simulink model "control_system"  (R2020b)
settings: Solver=FixedStepAuto  StartTime=0.0  StopTime=t_sim  FixedStep=Ts  RelTol=1e-2
values from neighbouring files (symbols this model uses):
  Hp = 10    [main_script.m]
  InitPosX = -2.4980e+03    (= -2498)    [main_script.m]
  InitPosY = -650.5503    [main_script.m]
  InitVelX = V0*cosd(InitYaw)    [main_script.m]
  InitVelY = V0*sind(InitYaw)    [main_script.m]
  InitYaw = 21    [main_script.m]
  lr = 1.592    [main_script.m]
  m = 1625    [main_script.m]
  Ts = 0.1    [main_script.m]
  V0 = 25    [main_script.m]
libraries: neural x856, simulink x1, autolibshared x1, drivingscenarioandsensors x1
(part 24 of 40)

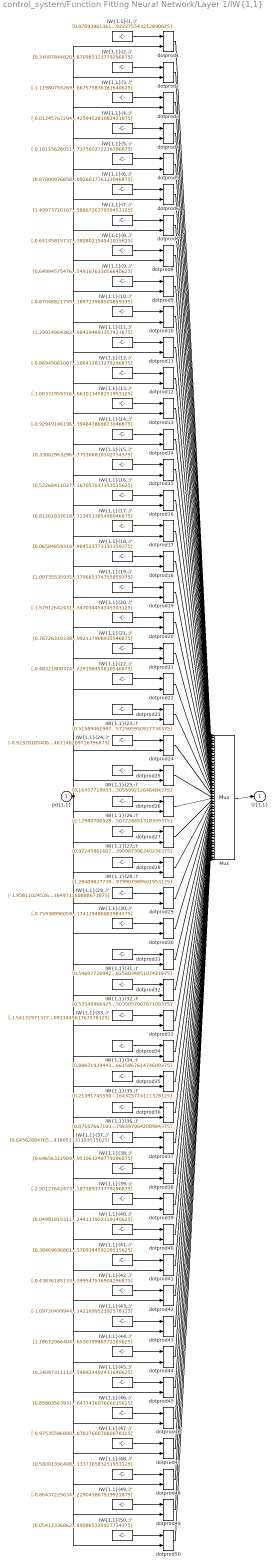
== system control_system/Function Fitting Neural Network/Layer 1/IW{1,1} ==
  "pd{1,1}" : Inport  PortDimensions=9  SampleTime=0.1
      mask Display: e = 0.06;c1 = [120 230 180]/255;c2 = ([120 230 180]+0)/(256+128);c3 = ([120 230 180]+128)/(256+128);patch([0 1 1 0],[0 0 1 1],c1);patch([0 1 1 1-e 1-e 0+e],[0 0 1 1-e 0+e 0+e],c2);patch([0 0 1 1-e 0+e 0+e],[0 1 1 1-e 1-e 0+e],c3);plot([0 1 1 0 0],[0 0 1 1 0]);
  "IW{1,1}(1,:)'" : Constant  Value=[0.97093961361378278152045595561503432691097259521484375;-0.28039871116987102883655325058498419821262359619140625;0.3851709807844587718506090823211707174777984619140625;-0.5135982842823201277582256807363592088222503662109375;1.1922160293525363439215425387374125421047210693359375;-2.639146237323939825358820598921738564968109130859375;-0.2450864019114529501752741680320468731224536895751953125;1.7910155270211147726655553924501873552799224853515625;-0.3880197795036404162516419091843999922275543212890625]
      mask Display: e = 0.06;c1 = [120 150 230]/255;c2 = ([120 150 230]+0)/383;c3 = ([120 150 230]+128)/383;patch([0 1 1 0],[0 0 1 1],c1);patch([0 1 1 1-e 1-e 0+e],[0 0 1 1-e 0+e 0+e],c2);patch([0 0 1 1-e 0+e 0+e],[0 1 1 1-e 1-e 0+e],c3);plot([0 1 1 0 0],[0 0 1 1 0]);disp('Weights');
  "IW{1,1}(10,:)'" : Constant  Value=[-0.87046821799074114434091598013765178620815277099609375;-0.270184812964925857858844437942025251686573028564453125;-0.43314155483321326034484854972106404602527618408203125;-1.590306799106527169129776666522957384586334228515625;-1.1862880482407736071337467365083284676074981689453125;-0.9888726559320486497739466358325444161891937255859375;-0.96914646726430786483064139247289858758449554443359375;-1.04056527906724483045763918198645114898681640625;-0.1494792541584611667015991542939445935189723968505859375]
      mask Display: e = 0.06;c1 = [120 150 230]/255;c2 = ([120 150 230]+0)/383;c3 = ([120 150 230]+128)/383;patch([0 1 1 0],[0 0 1 1],c1);patch([0 1 1 1-e 1-e 0+e],[0 0 1 1-e 0+e 0+e],c2);patch([0 0 1 1-e 0+e 0+e],[0 1 1 1-e 1-e 0+e],c3);plot([0 1 1 0 0],[0 0 1 1 0]);disp('Weights');
  "IW{1,1}(11,:)'" : Constant  Value=[1.2991496438276917135823396165505982935428619384765625;-0.25365900898659543560853535382193513214588165283203125;0.4141726146470963154655464677489362657070159912109375;1.210520214599590804738227234338410198688507080078125;-1.190198107523747328428953551338054239749908447265625;-1.869803133332969213853402834502048790454864501953125;-0.07196017006668704862892838036714238114655017852783203125;2.999680955949197258547656019800342619419097900390625;-0.059496514302423912645689796363512868992984294891357421875]
      mask Display: e = 0.06;c1 = [120 150 230]/255;c2 = ([120 150 230]+0)/383;c3 = ([120 150 230]+128)/383;patch([0 1 1 0],[0 0 1 1],c1);patch([0 1 1 1-e 1-e 0+e],[0 0 1 1-e 0+e 0+e],c2);patch([0 0 1 1-e 0+e 0+e],[0 1 1 1-e 1-e 0+e],c3);plot([0 1 1 0 0],[0 0 1 1 0]);disp('Weights');
  "IW{1,1}(12,:)'" : Constant  Value=[-0.86945061007791668572508569923229515552520751953125;0.290923752853725459122102847686619497835636138916015625;0.95093882023071019116144952931790612637996673583984375;-1.9489697439161499659121545846574008464813232421875;-1.519461066101597257471667035133577883243560791015625;1.2565348140057448489415037329308688640594482421875;0.933333136450000377948299501440487802028656005859375;1.0652420654480423412024947538156993687152862548828125;0.049200942200943502402576967824643361382186412811279296875]
      mask Display: e = 0.06;c1 = [120 150 230]/255;c2 = ([120 150 230]+0)/383;c3 = ([120 150 230]+128)/383;patch([0 1 1 0],[0 0 1 1],c1);patch([0 1 1 1-e 1-e 0+e],[0 0 1 1-e 0+e 0+e],c2);patch([0 0 1 1-e 0+e 0+e],[0 1 1 1-e 1-e 0+e],c3);plot([0 1 1 0 0],[0 0 1 1 0]);disp('Weights');
  "IW{1,1}(13,:)'" : Constant  Value=[-1.003319593162952827469780459068715572357177734375;0.67810826771338283958101555981556884944438934326171875;-0.61043188678200721586364352333475835621356964111328125;0.70916334762463384411290689968154765665531158447265625;-0.5759983806607589240655897810938768088817596435546875;2.2490521260628018040961251244880259037017822265625;0.72014281285539805121942436016979627311229705810546875;0.63362322182121577629487774174776859581470489501953125;-1.126765513624864656350155200925655663013458251953125]
      mask Display: e = 0.06;c1 = [120 150 230]/255;c2 = ([120 150 230]+0)/383;c3 = ([120 150 230]+128)/383;patch([0 1 1 0],[0 0 1 1],c1);patch([0 1 1 1-e 1-e 0+e],[0 0 1 1-e 0+e 0+e],c2);patch([0 0 1 1-e 0+e 0+e],[0 1 1 1-e 1-e 0+e],c3);plot([0 1 1 0 0],[0 0 1 1 0]);disp('Weights');
  "IW{1,1}(14,:)'" : Constant  Value=[-0.92949146196026521948851950583048164844512939453125;-1.1429665455757758163457538103102706372737884521484375;1.0519091572919772037408847609185613691806793212890625;-1.14525233529797532128213788382709026336669921875;-0.981528358989009586110796590219251811504364013671875;0.9179910649476141770719550549983978271484375;-1.318360733295090625460943556390702724456787109375;1.1479820287018203117668235790915787220001220703125;-0.44393580226848594616484433572622947394847869873046875]
      mask Display: e = 0.06;c1 = [120 150 230]/255;c2 = ([120 150 230]+0)/383;c3 = ([120 150 230]+128)/383;patch([0 1 1 0],[0 0 1 1],c1);patch([0 1 1 1-e 1-e 0+e],[0 0 1 1-e 0+e 0+e],c2);patch([0 0 1 1-e 0+e 0+e],[0 1 1 1-e 1-e 0+e],c3);plot([0 1 1 0 0],[0 0 1 1 0]);disp('Weights');
  "IW{1,1}(15,:)'" : Constant  Value=[0.338029632961837911420133195861126296222209930419921875;0.64599406331379516377211302824434824287891387939453125;0.83768969923422087475728403660468757152557373046875;0.1967697974008914829635585874711978249251842498779296875;1.222289857737168805584815345355309545993804931640625;0.408573274266887775940659821571898646652698516845703125;-1.3644966924852666156908753691823221743106842041015625;-0.63673533425992301371110215768567286431789398193359375;-0.438606434078379459062801970503642223775386810302734375]
      mask Display: e = 0.06;c1 = [120 150 230]/255;c2 = ([120 150 230]+0)/383;c3 = ([120 150 230]+128)/383;patch([0 1 1 0],[0 0 1 1],c1);patch([0 1 1 1-e 1-e 0+e],[0 0 1 1-e 0+e 0+e],c2);patch([0 0 1 1-e 0+e 0+e],[0 1 1 1-e 1-e 0+e],c3);plot([0 1 1 0 0],[0 0 1 1 0]);disp('Weights');
  "IW{1,1}(16,:)'" : Constant  Value=[0.52268411027939698509925392500008456408977508544921875;0.56795133558729860023817082037567161023616790771484375;-0.82591672355761158730302895492059178650379180908203125;-0.370849859231966172412597870788886211812496185302734375;-0.85030315566211955857767179622896946966648101806640625;-2.594022559460632759709142192150466144084930419921875;-1.1273055818606410038995591094135306775569915771484375;1.727361799815982923433921314426697790622711181640625;0.29135109056686714357198297875584103167057037353515625]
      mask Display: e = 0.06;c1 = [120 150 230]/255;c2 = ([120 150 230]+0)/383;c3 = ([120 150 230]+128)/383;patch([0 1 1 0],[0 0 1 1],c1);patch([0 1 1 1-e 1-e 0+e],[0 0 1 1-e 0+e 0+e],c2);patch([0 0 1 1-e 0+e 0+e],[0 1 1 1-e 1-e 0+e],c3);plot([0 1 1 0 0],[0 0 1 1 0]);disp('Weights');
  "IW{1,1}(17,:)'" : Constant  Value=[0.81261837618960386375732696251361630856990814208984375;0.11240683240479144855417104054140509106218814849853515625;-0.5429613049158803494975700232316739857196807861328125;-0.06735020182903361796178387521649710834026336669921875;0.39746836699794185765455267755896784365177154541015625;-2.289745303179948177074720661039464175701141357421875;-2.36823235121522213120215383241884410381317138671875;-0.01920417466123570948699494920219876803457736968994140625;-0.78248758849519528535410017866524867713451385498046875]
      mask Display: e = 0.06;c1 = [120 150 230]/255;c2 = ([120 150 230]+0)/383;c3 = ([120 150 230]+128)/383;patch([0 1 1 0],[0 0 1 1],c1);patch([0 1 1 1-e 1-e 0+e],[0 0 1 1-e 0+e 0+e],c2);patch([0 0 1 1-e 0+e 0+e],[0 1 1 1-e 1-e 0+e],c3);plot([0 1 1 0 0],[0 0 1 1 0]);disp('Weights');
  "IW{1,1}(18,:)'" : Constant  Value=[0.06584859319073210759398762093042023479938507080078125;0.62491571055994155070578699451289139688014984130859375;0.7990170181207203459194943206966854631900787353515625;-0.75432588489251550800673840058152563869953155517578125;0.13406440645860673299694099114276468753814697265625;-1.33187501082899029114514632965438067913055419921875;-0.1785974939056451937791081263640080578625202178955078125;1.7897623143730687633734532937523908913135528564453125;-1.1695125433076183352198995635262690484523773193359375]
      mask Display: e = 0.06;c1 = [120 150 230]/255;c2 = ([120 150 230]+0)/383;c3 = ([120 150 230]+128)/383;patch([0 1 1 0],[0 0 1 1],c1);patch([0 1 1 1-e 1-e 0+e],[0 0 1 1-e 0+e 0+e],c2);patch([0 0 1 1-e 0+e 0+e],[0 1 1 1-e 1-e 0+e],c3);plot([0 1 1 0 0],[0 0 1 1 0]);disp('Weights');
  "IW{1,1}(19,:)'" : Constant  Value=[1.0973553593516409687680379647645168006420135498046875;-0.57538307796085741419034320642822422087192535400390625;-0.6837986697134279534537881772848777472972869873046875;-0.94680710579524696157704966026358306407928466796875;0.88746712770898217303994215399143286049365997314453125;-1.381451882267370923074167876620776951313018798828125;1.0848135377034520132610850851051509380340576171875;0.261632884446667990374635337502695620059967041015625;-0.414726180288912116278510211486718617379665374755859375]
      mask Display: e = 0.06;c1 = [120 150 230]/255;c2 = ([120 150 230]+0)/383;c3 = ([120 150 230]+128)/383;patch([0 1 1 0],[0 0 1 1],c1);patch([0 1 1 1-e 1-e 0+e],[0 0 1 1-e 0+e 0+e],c2);patch([0 0 1 1-e 0+e 0+e],[0 1 1 1-e 1-e 0+e],c3);plot([0 1 1 0 0],[0 0 1 1 0]);disp('Weights');
  "IW{1,1}(2,:)'" : Constant  Value=[0.340078448202071947914504335130914114415645599365234375;0.61152168668360207259837579840677790343761444091796875;1.1084410511733011617252486757934093475341796875;-0.62989834861553595235506008975789882242679595947265625;-0.58042049387658967152248123966273851692676544189453125;-2.466934744743214391604624324827454984188079833984375;-1.2023642587252083568927218948374502360820770263671875;1.0666891089756165289514910909929312765598297119140625;-0.5594774025453748134140141701209358870983123779296875]
      mask Display: e = 0.06;c1 = [120 150 230]/255;c2 = ([120 150 230]+0)/383;c3 = ([120 150 230]+128)/383;patch([0 1 1 0],[0 0 1 1],c1);patch([0 1 1 1-e 1-e 0+e],[0 0 1 1-e 0+e 0+e],c2);patch([0 0 1 1-e 0+e 0+e],[0 1 1 1-e 1-e 0+e],c3);plot([0 1 1 0 0],[0 0 1 1 0]);disp('Weights');
  "IW{1,1}(20,:)'" : Constant  Value=[-1.57912642431413541288520718808285892009735107421875;0.61409549742207769629231961516779847443103790283203125;1.1686478953490155863192967444774694740772247314453125;-1.1848793747106174389926991352695040404796600341796875;-1.239529920774651738923921584500931203365325927734375;1.809648206205790810230382703593932092189788818359375;-0.20529698998786205521582814981229603290557861328125;3.47991716679978413395701863919384777545928955078125;-0.1594062963675073885116972860487294383347034454345703125]
      mask Display: e = 0.06;c1 = [120 150 230]/255;c2 = ([120 150 230]+0)/383;c3 = ([120 150 230]+128)/383;patch([0 1 1 0],[0 0 1 1],c1);patch([0 1 1 1-e 1-e 0+e],[0 0 1 1-e 0+e 0+e],c2);patch([0 0 1 1-e 0+e 0+e],[0 1 1 1-e 1-e 0+e],c3);plot([0 1 1 0 0],[0 0 1 1 0]);disp('Weights');
  "IW{1,1}(21,:)'" : Constant  Value=[0.7672631033851498028042215082678012549877166748046875;-0.458108958975613156372475032185320742428302764892578125;-0.59701861006420475774802980595268309116363525390625;-0.519756145505974931353421197854913771152496337890625;0.54766554871049688557604895322583615779876708984375;2.312553685817124726753490904229693114757537841796875;0.11270256966186241454064287381697795353829860687255859375;-1.7338209275897338290661764403921552002429962158203125;-0.26046106414641723159064667925122193992137908935546875]
      mask Display: e = 0.06;c1 = [120 150 230]/255;c2 = ([120 150 230]+0)/383;c3 = ([120 150 230]+128)/383;patch([0 1 1 0],[0 0 1 1],c1);patch([0 1 1 1-e 1-e 0+e],[0 0 1 1-e 0+e 0+e],c2);patch([0 0 1 1-e 0+e 0+e],[0 1 1 1-e 1-e 0+e],c3);plot([0 1 1 0 0],[0 0 1 1 0]);disp('Weights');
  "IW{1,1}(22,:)'" : Constant  Value=[-0.48321808374106300920658441100385971367359161376953125;-0.65067428012154138183831264541368000209331512451171875;0.403709011817810381472781955380924046039581298828125;-0.97435270094193315859598669703700579702854156494140625;0.94881194703902094200742567409179173409938812255859375;-0.3906213358896533094366532168351113796234130859375;-0.477089342851166831049880556747666560113430023193359375;1.0488331207768648578593229103717021644115447998046875;1.275361389429331193667849220219068229198455810546875]
      mask Display: e = 0.06;c1 = [120 150 230]/255;c2 = ([120 150 230]+0)/383;c3 = ([120 150 230]+128)/383;patch([0 1 1 0],[0 0 1 1],c1);patch([0 1 1 1-e 1-e 0+e],[0 0 1 1-e 0+e 0+e],c2);patch([0 0 1 1-e 0+e 0+e],[0 1 1 1-e 1-e 0+e],c3);plot([0 1 1 0 0],[0 0 1 1 0]);disp('Weights');
  "IW{1,1}(23,:)'" : Constant  Value=[0.51589461997649888047590138739906251430511474609375;0.87745139464428933973039193006115965545177459716796875;-0.032613147418183031922556125437040464021265506744384765625;-0.03530138783985899142425779473342117853462696075439453125;1.190955473178289647506744586280547082424163818359375;2.559180139348819604805385097279213368892669677734375;0.1537049497733080360983848322575795464217662811279296875;1.8488371095364704022045998499379493296146392822265625;0.82838062523518285473755895509384572505950927734375]
      mask Display: e = 0.06;c1 = [120 150 230]/255;c2 = ([120 150 230]+0)/383;c3 = ([120 150 230]+128)/383;patch([0 1 1 0],[0 0 1 1],c1);patch([0 1 1 1-e 1-e 0+e],[0 0 1 1-e 0+e 0+e],c2);patch([0 0 1 1-e 0+e 0+e],[0 1 1 1-e 1-e 0+e],c3);plot([0 1 1 0 0],[0 0 1 1 0]);disp('Weights');
  "IW{1,1}(24,:)'" : Constant  Value=[-0.92320185406252708304464249522425234317779541015625;0.1589026907972997670892567612099810503423213958740234375;1.336759816706434289557137162773869931697845458984375;-0.5072895852030858687697900677449069917201995849609375;-0.83277156532756346773993527676793746650218963623046875;-0.58680259947876234338792755806935019791126251220703125;0.98203138856916927235118919270462356507778167724609375;0.1387309905135986343172049828353920020163059234619140625;-1.498732567071687338255969734746031463146209716796875]
      mask Display: e = 0.06;c1 = [120 150 230]/255;c2 = ([120 150 230]+0)/383;c3 = ([120 150 230]+128)/383;patch([0 1 1 0],[0 0 1 1],c1);patch([0 1 1 1-e 1-e 0+e],[0 0 1 1-e 0+e 0+e],c2);patch([0 0 1 1-e 0+e 0+e],[0 1 1 1-e 1-e 0+e],c3);plot([0 1 1 0 0],[0 0 1 1 0]);disp('Weights');
  "IW{1,1}(25,:)'" : Constant  Value=[0.164577189330164352920604642349644564092159271240234375;0.84274510322094287051442051961203105747699737548828125;1.0828171979316782991276113534695468842983245849609375;-0.95362354157796136444602552728611044585704803466796875;-0.65823826889210146351416597099159844219684600830078125;-0.342232460185585007916841959740850143134593963623046875;-1.31956634967429931037941059912554919719696044921875;-1.3632672320762908579894201466231606900691986083984375;-0.58440502948554795548119500381289981305599212646484375]
      mask Display: e = 0.06;c1 = [120 150 230]/255;c2 = ([120 150 230]+0)/383;c3 = ([120 150 230]+128)/383;patch([0 1 1 0],[0 0 1 1],c1);patch([0 1 1 1-e 1-e 0+e],[0 0 1 1-e 0+e 0+e],c2);patch([0 0 1 1-e 0+e 0+e],[0 1 1 1-e 1-e 0+e],c3);plot([0 1 1 0 0],[0 0 1 1 0]);disp('Weights');
  "IW{1,1}(26,:)'" : Constant  Value=[2.129807065288331191510451390058733522891998291015625;-0.107603565378774523875193835920072160661220550537109375;0.3974472819784342636495466649648733437061309814453125;0.2283305403113514431279185146195231936872005462646484375;-1.17135151038194607053810614161193370819091796875;-0.09955161999984911413985599892839672975242137908935546875;-0.69388861218623343329880981400492601096630096435546875;1.5917799632123525999105595474247820675373077392578125;0.07577917958936251918711235475711873732507228851318359375]
      mask Display: e = 0.06;c1 = [120 150 230]/255;c2 = ([120 150 230]+0)/383;c3 = ([120 150 230]+128)/383;patch([0 1 1 0],[0 0 1 1],c1);patch([0 1 1 1-e 1-e 0+e],[0 0 1 1-e 0+e 0+e],c2);patch([0 0 1 1-e 0+e 0+e],[0 1 1 1-e 1-e 0+e],c3);plot([0 1 1 0 0],[0 0 1 1 0]);disp('Weights');
  "IW{1,1}(27,:)'" : Constant  Value=[0.972458616076971704700326881720684468746185302734375;0.80071168334724396320467576515511609613895416259765625;-0.69820535755774570940701551080564968287944793701171875;-0.5759124849266401557912331554689444601535797119140625;-0.128118934045561239098987016404862515628337860107421875;-1.478205651886735250144511155667714774608612060546875;0.0077068368952901457336057688962682732380926609039306640625;-0.998042389125082696210711219464428722858428955078125;-0.714100168764340903493348378106020390987396240234375]
      mask Display: e = 0.06;c1 = [120 150 230]/255;c2 = ([120 150 230]+0)/383;c3 = ([120 150 230]+128)/383;patch([0 1 1 0],[0 0 1 1],c1);patch([0 1 1 1-e 1-e 0+e],[0 0 1 1-e 0+e 0+e],c2);patch([0 0 1 1-e 0+e 0+e],[0 1 1 1-e 1-e 0+e],c3);plot([0 1 1 0 0],[0 0 1 1 0]);disp('Weights');
  "IW{1,1}(28,:)'" : Constant  Value=[1.2940982773928013660480473845382221043109893798828125;-0.375899268560394850258177257273928262293338775634765625;0.52795145605138327216110383233171887695789337158203125;0.8920181642611628713979143867618404328823089599609375;-0.7564801989411666927054511688766069710254669189453125;-0.93565270712781833939430953250848688185214996337890625;1.2753434908208323150802243617363274097442626953125;-2.1016583865335274339258830877952277660369873046875;-0.96344937374039407718129268687334842979907989501953125]
      mask Display: e = 0.06;c1 = [120 150 230]/255;c2 = ([120 150 230]+0)/383;c3 = ([120 150 230]+128)/383;patch([0 1 1 0],[0 0 1 1],c1);patch([0 1 1 1-e 1-e 0+e],[0 0 1 1-e 0+e 0+e],c2);patch([0 0 1 1-e 0+e 0+e],[0 1 1 1-e 1-e 0+e],c3);plot([0 1 1 0 0],[0 0 1 1 0]);disp('Weights');
  "IW{1,1}(29,:)'" : Constant  Value=[-1.9581102452695378079994270592578686773777008056640625;-0.51412525497394268025885821771225892007350921630859375;0.20836627953751907238455487458850257098674774169921875;-0.67867145203121570506965554159251041710376739501953125;-0.73024135157208525104266527705476619303226470947265625;-1.352942975596346020239479912561364471912384033203125;0.396568187054604115449052414987818337976932525634765625;1.317863646844906089228288692538626492023468017578125;-1.97243397611674264879866314004175364971160888671875]
      mask Display: e = 0.06;c1 = [120 150 230]/255;c2 = ([120 150 230]+0)/383;c3 = ([120 150 230]+128)/383;patch([0 1 1 0],[0 0 1 1],c1);patch([0 1 1 1-e 1-e 0+e],[0 0 1 1-e 0+e 0+e],c2);patch([0 0 1 1-e 0+e 0+e],[0 1 1 1-e 1-e 0+e],c3);plot([0 1 1 0 0],[0 0 1 1 0]);disp('Weights');
  "IW{1,1}(3,:)'" : Constant  Value=[-1.1198075526975130866702556886593811213970184326171875;-0.20507969346321497372542808079742826521396636962890625;-0.289346350572056376648788500460796058177947998046875;0.720249732554860688793496592552401125431060791015625;-0.331892783688242765105513853995944373309612274169921875;-1.233167629340175874830265456694178283214569091796875;0.6903163444130335779647111849044449627399444580078125;-0.347081239760978821351500300806947052478790283203125;0.90246068479395946670962302960106171667575836181640625]
      mask Display: e = 0.06;c1 = [120 150 230]/255;c2 = ([120 150 230]+0)/383;c3 = ([120 150 230]+128)/383;patch([0 1 1 0],[0 0 1 1],c1);patch([0 1 1 1-e 1-e 0+e],[0 0 1 1-e 0+e 0+e],c2);patch([0 0 1 1-e 0+e 0+e],[0 1 1 1-e 1-e 0+e],c3);plot([0 1 1 0 0],[0 0 1 1 0]);disp('Weights');
  "IW{1,1}(30,:)'" : Constant  Value=[-0.759389960599416991016141764703206717967987060546875;0.2840216328908475862391469490830786526203155517578125;0.94276840524974547808056968278833664953708648681640625;0.97160631832165711418980436064884997904300689697265625;-0.58575567778431592014243278754292987287044525146484375;0.8372478811272221488337663686252199113368988037109375;-0.71782872175648304580164449362200684845447540283203125;-0.436041221124511102491538849790231324732303619384765625;1.1028566606177123698984132715850137174129486083984375]
      mask Display: e = 0.06;c1 = [120 150 230]/255;c2 = ([120 150 230]+0)/383;c3 = ([120 150 230]+128)/383;patch([0 1 1 0],[0 0 1 1],c1);patch([0 1 1 1-e 1-e 0+e],[0 0 1 1-e 0+e 0+e],c2);patch([0 0 1 1-e 0+e 0+e],[0 1 1 1-e 1-e 0+e],c3);plot([0 1 1 0 0],[0 0 1 1 0]);disp('Weights');
  "IW{1,1}(31,:)'" : Constant  Value=[0.5460772094207744231653123279102146625518798828125;0.460953363760126411108331012655980885028839111328125;-0.2115703979530784983875690841159666888415813446044921875;0.69504683404170808369570977447438053786754608154296875;0.8940914594258568826035116217099130153656005859375;-1.1341484239892289931361801791354082524776458740234375;-0.78412324798395693914443427274818532168865203857421875;0.458013400742934617682067255373112857341766357421875;-0.87559191277812054021723042751546017825603485107421875]
      mask Display: e = 0.06;c1 = [120 150 230]/255;c2 = ([120 150 230]+0)/383;c3 = ([120 150 230]+128)/383;patch([0 1 1 0],[0 0 1 1],c1);patch([0 1 1 1-e 1-e 0+e],[0 0 1 1-e 0+e 0+e],c2);patch([0 0 1 1-e 0+e 0+e],[0 1 1 1-e 1-e 0+e],c3);plot([0 1 1 0 0],[0 0 1 1 0]);disp('Weights');
  "IW{1,1}(32,:)'" : Constant  Value=[0.5354996642529721295744593589915893971920013427734375;1.2428883524386815651041615637950599193572998046875;0.228676873276494274644932147566578350961208343505859375;-0.74924171147733920061995149808353744447231292724609375;-0.16774896417198348341770497427205555140972137451171875;-0.196043865385012450186508203842095099389553070068359375;0.91169744811784669824561433415510691702365875244140625;2.152452022970312128791192662902176380157470703125;-0.6080750191048698294338237246847711503505706787109375]
      mask Display: e = 0.06;c1 = [120 150 230]/255;c2 = ([120 150 230]+0)/383;c3 = ([120 150 230]+128)/383;patch([0 1 1 0],[0 0 1 1],c1);patch([0 1 1 1-e 1-e 0+e],[0 0 1 1-e 0+e 0+e],c2);patch([0 0 1 1-e 0+e 0+e],[0 1 1 1-e 1-e 0+e],c3);plot([0 1 1 0 0],[0 0 1 1 0]);disp('Weights');
  "IW{1,1}(33,:)'" : Constant  Value=[-1.54132971377970395820966587052680552005767822265625;-0.25072633293704693624448509581270627677440643310546875;0.159123795845034277096630148662370629608631134033203125;0.842653609044052398502344658481888473033905029296875;-0.10573959777820692018668324863028828985989093780517578125;-0.032706632404859485585557621334373834542930126190185546875;1.010366189247158263952997003798373043537139892578125;0.59077516492751780408099193664384074509143829345703125;-1.4585530146121705730166695502703078091144561767578125]
      mask Display: e = 0.06;c1 = [120 150 230]/255;c2 = ([120 150 230]+0)/383;c3 = ([120 150 230]+128)/383;patch([0 1 1 0],[0 0 1 1],c1);patch([0 1 1 1-e 1-e 0+e],[0 0 1 1-e 0+e 0+e],c2);patch([0 0 1 1-e 0+e 0+e],[0 1 1 1-e 1-e 0+e],c3);plot([0 1 1 0 0],[0 0 1 1 0]);disp('Weights');
  "IW{1,1}(34,:)'" : Constant  Value=[0.88671928443622871629514747837674804031848907470703125;-0.120878905322355512108600805731839500367641448974609375;-0.4035700109378390632031141649349592626094818115234375;-0.92663839697876160261813538454589433968067169189453125;-1.0135453088708319402400093167671002447605133056640625;-1.173695312179412919562082606717012822628021240234375;-0.5347377780826312321238447111682035028934478759765625;0.127868778308200814475270590264699421823024749755859375;0.91237645222570085135060935499495826661586761474609375]
      mask Display: e = 0.06;c1 = [120 150 230]/255;c2 = ([120 150 230]+0)/383;c3 = ([120 150 230]+128)/383;patch([0 1 1 0],[0 0 1 1],c1);patch([0 1 1 1-e 1-e 0+e],[0 0 1 1-e 0+e 0+e],c2);patch([0 0 1 1-e 0+e 0+e],[0 1 1 1-e 1-e 0+e],c3);plot([0 1 1 0 0],[0 0 1 1 0]);disp('Weights');
  "IW{1,1}(35,:)'" : Constant  Value=[0.2139174555065020688626731271142489276826381683349609375;-0.94378848270968995759488961994065903127193450927734375;-0.77573954351650609151391790874185971915721893310546875;0.832673531343797179715693346224725246429443359375;0.5534326111105565271230943835689686238765716552734375;0.483365499823072308771543248440138995647430419921875;-1.0535779933159463706004999039578251540660858154296875;0.1461396229710316685412863080273382365703582763671875;-1.2308373766330504839316972720553167164325714111328125]
      mask Display: e = 0.06;c1 = [120 150 230]/255;c2 = ([120 150 230]+0)/383;c3 = ([120 150 230]+128)/383;patch([0 1 1 0],[0 0 1 1],c1);patch([0 1 1 1-e 1-e 0+e],[0 0 1 1-e 0+e 0+e],c2);patch([0 0 1 1-e 0+e 0+e],[0 1 1 1-e 1-e 0+e],c3);plot([0 1 1 0 0],[0 0 1 1 0]);disp('Weights');
  "IW{1,1}(36,:)'" : Constant  Value=[0.071076671037090921601020454545505344867706298828125;0.664168033627640763683075419976375997066497802734375;1.8291748250620083471318366719060577452182769775390625;0.3820678757705116002085787840769626200199127197265625;0.59425875284591211933360455077490769326686859130859375;-0.76784223084368019573986430259537883102893829345703125;-0.655048484051070634137658998952247202396392822265625;-2.145149871234647509510296004009433090686798095703125;-1.4557464670865216671558073358028195798397064208984375]
      mask Display: e = 0.06;c1 = [120 150 230]/255;c2 = ([120 150 230]+0)/383;c3 = ([120 150 230]+128)/383;patch([0 1 1 0],[0 0 1 1],c1);patch([0 1 1 1-e 1-e 0+e],[0 0 1 1-e 0+e 0+e],c2);patch([0 0 1 1-e 0+e 0+e],[0 1 1 1-e 1-e 0+e],c3);plot([0 1 1 0 0],[0 0 1 1 0]);disp('Weights');
  "IW{1,1}(37,:)'" : Constant  Value=[0.6456288476568701195645871848682872951030731201171875;-0.65799923001170046443775163425016216933727264404296875;0.311582392682186404275768154548131860792636871337890625;-0.89148107540302323759107139267143793404102325439453125;-0.50996951927726552611375154810957610607147216796875;-0.51393130227626360184700615718611516058444976806640625;1.078650466544016861547561347833834588527679443359375;-0.73422117746091630774429859229712747037410736083984375;-0.95155828196638891913750057938159443438053131103515625]
      mask Display: e = 0.06;c1 = [120 150 230]/255;c2 = ([120 150 230]+0)/383;c3 = ([120 150 230]+128)/383;patch([0 1 1 0],[0 0 1 1],c1);patch([0 1 1 1-e 1-e 0+e],[0 0 1 1-e 0+e 0+e],c2);patch([0 0 1 1-e 0+e 0+e],[0 1 1 1-e 1-e 0+e],c3);plot([0 1 1 0 0],[0 0 1 1 0]);disp('Weights');
  "IW{1,1}(38,:)'" : Constant  Value=[0.6965632290952339378264923652750439941883087158203125;-1.047869280408078029864782365621067583560943603515625;0.10172333557136960247024859427256160415709018707275390625;-0.65579721068447904830378547558211721479892730712890625;0.476182384031906769106257115709013305604457855224609375;-0.454386696705189108147493470823974348604679107666015625;-0.67927572398451141477693226988776586949825286865234375;-0.9500830060727418757693385487073101103305816650390625;1.5277450016389397813298955952632240951061248779296875]
      mask Display: e = 0.06;c1 = [120 150 230]/255;c2 = ([120 150 230]+0)/383;c3 = ([120 150 230]+128)/383;patch([0 1 1 0],[0 0 1 1],c1);patch([0 1 1 1-e 1-e 0+e],[0 0 1 1-e 0+e 0+e],c2);patch([0 0 1 1-e 0+e 0+e],[0 1 1 1-e 1-e 0+e],c3);plot([0 1 1 0 0],[0 0 1 1 0]);disp('Weights');
  "IW{1,1}(39,:)'" : Constant  Value=[-2.501276424736501358125906335772015154361724853515625;-1.54408584292858819253524416126310825347900390625;0.53902133932544804562070339670754037797451019287109375;-2.47586042911307036007428905577398836612701416015625;-1.58608884985863429761820952990092337131500244140625;-1.8602628445853326422110285420785658061504364013671875;-0.79149527778107697795206831870018504559993743896484375;0.52007634687461756772819398975116200745105743408203125;0.65448293706638682731835388040053658187389373779296875]
      mask Display: e = 0.06;c1 = [120 150 230]/255;c2 = ([120 150 230]+0)/383;c3 = ([120 150 230]+128)/383;patch([0 1 1 0],[0 0 1 1],c1);patch([0 1 1 1-e 1-e 0+e],[0 0 1 1-e 0+e 0+e],c2);patch([0 0 1 1-e 0+e 0+e],[0 1 1 1-e 1-e 0+e],c3);plot([0 1 1 0 0],[0 0 1 1 0]);disp('Weights');
  "IW{1,1}(4,:)'" : Constant  Value=[-0.01245767294369288895328207189550084876827895641326904296875;-0.411636498589336874420752110381727106869220733642578125;0.2343696751666357325216694107439252547919750213623046875;0.151189163508950119574336667938041500747203826904296875;-0.55434305624034874160344088522833772003650665283203125;-1.8245528196456344272036176334950141608715057373046875;-0.463261564773732870126110583441914059221744537353515625;1.46145194046994930658911471255123615264892578125;2.084219744558360343233971434528939425945281982421875]
      mask Display: e = 0.06;c1 = [120 150 230]/255;c2 = ([120 150 230]+0)/383;c3 = ([120 150 230]+128)/383;patch([0 1 1 0],[0 0 1 1],c1);patch([0 1 1 1-e 1-e 0+e],[0 0 1 1-e 0+e 0+e],c2);patch([0 0 1 1-e 0+e 0+e],[0 1 1 1-e 1-e 0+e],c3);plot([0 1 1 0 0],[0 0 1 1 0]);disp('Weights');
  "IW{1,1}(40,:)'" : Constant  Value=[0.0499181531106483167281595569875207729637622833251953125;1.0051321772202594928558028186671435832977294921875;-0.270173244365803422173399894745671190321445465087890625;-1.3445729513710948932470046202070079743862152099609375;-0.2261562490857440266278644003250519745051860809326171875;1.9768896600832850385387473579612560570240020751953125;-0.96232631804396728814054995382321067154407501220703125;0.251580362866357931661553948288201354444026947021484375;1.15310724398443031901706490316428244113922119140625]
      mask Display: e = 0.06;c1 = [120 150 230]/255;c2 = ([120 150 230]+0)/383;c3 = ([120 150 230]+128)/383;patch([0 1 1 0],[0 0 1 1],c1);patch([0 1 1 1-e 1-e 0+e],[0 0 1 1-e 0+e 0+e],c2);patch([0 0 1 1-e 0+e 0+e],[0 1 1 1-e 1-e 0+e],c3);plot([0 1 1 0 0],[0 0 1 1 0]);disp('Weights');
  "IW{1,1}(41,:)'" : Constant  Value=[0.38469696861631141882043039004202000796794891357421875;-0.2480663135903987959185457157218479551374912261962890625;-1.1349625028722438724315679792198352515697479248046875;-0.7068117105996154503344541808473877608776092529296875;1.0943346055495497548548655686317943036556243896484375;0.217780452520371980984492665811558254063129425048828125;-0.8727094143813707294299319983110763132572174072265625;0.63296503258427627702786821828340180218219757080078125;0.30266956728881366789352114210487343370914459228515625]
      mask Display: e = 0.06;c1 = [120 150 230]/255;c2 = ([120 150 230]+0)/383;c3 = ([120 150 230]+128)/383;patch([0 1 1 0],[0 0 1 1],c1);patch([0 1 1 1-e 1-e 0+e],[0 0 1 1-e 0+e 0+e],c2);patch([0 0 1 1-e 0+e 0+e],[0 1 1 1-e 1-e 0+e],c3);plot([0 1 1 0 0],[0 0 1 1 0]);disp('Weights');
  "IW{1,1}(42,:)'" : Constant  Value=[-0.4383618513340941102995884648407809436321258544921875;-0.57418463271939013115030547851347364485263824462890625;-0.66654353817884282040751031672698445618152618408203125;-0.28523372835698623806166551730711944401264190673828125;0.97122275204309260754342858490417711436748504638671875;0.53016822367742044708194271152024157345294952392578125;-0.5308267262522157192705662964726798236370086669921875;-1.204748771676599883306835181429050862789154052734375;0.52152863773203594899285917563247494399547576904296875]
      mask Display: e = 0.06;c1 = [120 150 230]/255;c2 = ([120 150 230]+0)/383;c3 = ([120 150 230]+128)/383;patch([0 1 1 0],[0 0 1 1],c1);patch([0 1 1 1-e 1-e 0+e],[0 0 1 1-e 0+e 0+e],c2);patch([0 0 1 1-e 0+e 0+e],[0 1 1 1-e 1-e 0+e],c3);plot([0 1 1 0 0],[0 0 1 1 0]);disp('Weights');
  "IW{1,1}(43,:)'" : Constant  Value=[-1.097204999444521877904890061472542583942413330078125;-0.06095196396622311330038002097353455610573291778564453125;-1.2088855521526815639532514978782273828983306884765625;-0.5664032353071044578740611541434191167354583740234375;1.039673180341422753514279975206591188907623291015625;-1.90933576109207781001941839349456131458282470703125;0.55569237221125933334775481853284873068332672119140625;-0.425995643434998016996217984342365525662899017333984375;-0.032752510386764743799403731827624142169952392578125]
      mask Display: e = 0.06;c1 = [120 150 230]/255;c2 = ([120 150 230]+0)/383;c3 = ([120 150 230]+128)/383;patch([0 1 1 0],[0 0 1 1],c1);patch([0 1 1 1-e 1-e 0+e],[0 0 1 1-e 0+e 0+e],c2);patch([0 0 1 1-e 0+e 0+e],[0 1 1 1-e 1-e 0+e],c3);plot([0 1 1 0 0],[0 0 1 1 0]);disp('Weights');
  "IW{1,1}(44,:)'" : Constant  Value=[1.1867206640414227347690712122130207717418670654296875;-0.51641328540057163110077453893609344959259033203125;-1.029288781821291909324145308346487581729888916015625;0.1761470882763403189574802354400162585079669952392578125;-0.817240127933413607053125815582461655139923095703125;-0.29719985756557354417140004443353973329067230224609375;-0.376403083287819573143906382028944790363311767578125;0.7379027639523181303360388483270071446895599365234375;0.522499458097746671825234443531371653079986572265625]
      mask Display: e = 0.06;c1 = [120 150 230]/255;c2 = ([120 150 230]+0)/383;c3 = ([120 150 230]+128)/383;patch([0 1 1 0],[0 0 1 1],c1);patch([0 1 1 1-e 1-e 0+e],[0 0 1 1-e 0+e 0+e],c2);patch([0 0 1 1-e 0+e 0+e],[0 1 1 1-e 1-e 0+e],c3);plot([0 1 1 0 0],[0 0 1 1 0]);disp('Weights');
  "IW{1,1}(45,:)'" : Constant  Value=[0.240973111125132255505576495124842040240764617919921875;0.377473013572193483167183103432762436568737030029296875;0.416452240351548874652820586561574600636959075927734375;-0.166501497516372831686481958968215622007846832275390625;-1.834082844585235960721547598950564861297607421875;3.3892664252582758166454368620179593563079833984375;-0.0748724992258840982284340270780376158654689788818359375;-0.444894164332242880721679512134869582951068878173828125;-0.14343269040447526041504033855744637548923492431640625]
      mask Display: e = 0.06;c1 = [120 150 230]/255;c2 = ([120 150 230]+0)/383;c3 = ([120 150 230]+128)/383;patch([0 1 1 0],[0 0 1 1],c1);patch([0 1 1 1-e 1-e 0+e],[0 0 1 1-e 0+e 0+e],c2);patch([0 0 1 1-e 0+e 0+e],[0 1 1 1-e 1-e 0+e],c3);plot([0 1 1 0 0],[0 0 1 1 0]);disp('Weights');
  "IW{1,1}(46,:)'" : Constant  Value=[0.85803563931209880788486543679027818143367767333984375;-0.63961669920042718562314121300005353987216949462890625;-1.8790915052350367631106564658693969249725341796875;-0.124242937280011067624485576743609271943569183349609375;0.434112243372880957092974085753667168319225311279296875;-0.07580442069907462887545790408694301731884479522705078125;-0.20038215540647164036869298797682859003543853759765625;-0.4380871196766673580924589259666390717029571533203125;0.404227687614099606694395561135024763643741607666015625]
      mask Display: e = 0.06;c1 = [120 150 230]/255;c2 = ([120 150 230]+0)/383;c3 = ([120 150 230]+128)/383;patch([0 1 1 0],[0 0 1 1],c1);patch([0 1 1 1-e 1-e 0+e],[0 0 1 1-e 0+e 0+e],c2);patch([0 0 1 1-e 0+e 0+e],[0 1 1 1-e 1-e 0+e],c3);plot([0 1 1 0 0],[0 0 1 1 0]);disp('Weights');
  "IW{1,1}(47,:)'" : Constant  Value=[-0.97535586890674874638307301211170852184295654296875;-0.299335465871109318580778335672221146523952484130859375;-0.28790071651083148918104370750370435416698455810546875;-1.707306349052662763909893328673206269741058349609375;-0.424632458065148321590953628401621244847774505615234375;-1.7167520343473963162495010692509822547435760498046875;-1.3155488353961513059431354122352786362171173095703125;-0.73148446576655212769679792472743429243564605712890625;-0.90745028209644396088862094984506256878376007080078125]
      mask Display: e = 0.06;c1 = [120 150 230]/255;c2 = ([120 150 230]+0)/383;c3 = ([120 150 230]+128)/383;patch([0 1 1 0],[0 0 1 1],c1);patch([0 1 1 1-e 1-e 0+e],[0 0 1 1-e 0+e 0+e],c2);patch([0 0 1 1-e 0+e 0+e],[0 1 1 1-e 1-e 0+e],c3);plot([0 1 1 0 0],[0 0 1 1 0]);disp('Weights');
  "IW{1,1}(48,:)'" : Constant  Value=[0.58001396408077654509582998798578046262264251708984375;-1.519046330984501924632468217168934643268585205078125;-0.56950056035899765394248106531449593603610992431640625;0.324523052716408189066754630403011105954647064208984375;-1.27647180417102301674958653165958821773529052734375;0.77654160714141429178170028535532765090465545654296875;0.65278250713822616457804315359680913388729095458984375;0.71456416558735924571266195926000364124774932861328125;0.96951647422195297298941341068712063133716583251953125]
      mask Display: e = 0.06;c1 = [120 150 230]/255;c2 = ([120 150 230]+0)/383;c3 = ([120 150 230]+128)/383;patch([0 1 1 0],[0 0 1 1],c1);patch([0 1 1 1-e 1-e 0+e],[0 0 1 1-e 0+e 0+e],c2);patch([0 0 1 1-e 0+e 0+e],[0 1 1 1-e 1-e 0+e],c3);plot([0 1 1 0 0],[0 0 1 1 0]);disp('Weights');
  "IW{1,1}(49,:)'" : Constant  Value=[-0.86437225634516712258204051977372728288173675537109375;0.98171685428277866147794838980189524590969085693359375;0.019456189134307556865000066181892179884016513824462890625;0.93457076825025009458869362788391299545764923095703125;-0.716132009219719645187751666526310145854949951171875;0.1391102844191524356975975251771160401403903961181640625;0.6054396940132116267108131069107912480831146240234375;0.97250202007511610258205791978980414569377899169921875;0.479736723293402611556501824452425353229045867919921875]
      mask Display: e = 0.06;c1 = [120 150 230]/255;c2 = ([120 150 230]+0)/383;c3 = ([120 150 230]+128)/383;patch([0 1 1 0],[0 0 1 1],c1);patch([0 1 1 1-e 1-e 0+e],[0 0 1 1-e 0+e 0+e],c2);patch([0 0 1 1-e 0+e 0+e],[0 1 1 1-e 1-e 0+e],c3);plot([0 1 1 0 0],[0 0 1 1 0]);disp('Weights');
  "IW{1,1}(5,:)'" : Constant  Value=[-0.181156260513459788086265689344145357608795166015625;0.6201558592768481315005146825569681823253631591796875;-0.92873871939931651464661399586475454270839691162109375;-0.14649962329492416390763764866278506815433502197265625;-0.723763893029772287235346084344200789928436279296875;-0.175056695761272529399121822279994376003742218017578125;-1.1039947092468300748890897011733613908290863037109375;0.84960381390248074229276653568376787006855010986328125;-0.72889227291211244885715814234572462737560272216796875]
      mask Display: e = 0.06;c1 = [120 150 230]/255;c2 = ([120 150 230]+0)/383;c3 = ([120 150 230]+128)/383;patch([0 1 1 0],[0 0 1 1],c1);patch([0 1 1 1-e 1-e 0+e],[0 0 1 1-e 0+e 0+e],c2);patch([0 0 1 1-e 0+e 0+e],[0 1 1 1-e 1-e 0+e],c3);plot([0 1 1 0 0],[0 0 1 1 0]);disp('Weights');
  "IW{1,1}(50,:)'" : Constant  Value=[0.054123368625048372260177842463235720060765743255615234375;0.74976423299714334280707817015354521572589874267578125;-1.1783432860728193514177064571413211524486541748046875;-0.69060360291757250106314813820063136518001556396484375;0.86871111050459293156933426871546544134616851806640625;-0.406972539882097306129793423679075203835964202880859375;0.031903777161261158423766204350613406859338283538818359375;0.56555808722542566524538187877624295651912689208984375;-1.14937646256341707839965238235890865325927734375]
      mask Display: e = 0.06;c1 = [120 150 230]/255;c2 = ([120 150 230]+0)/383;c3 = ([120 150 230]+128)/383;patch([0 1 1 0],[0 0 1 1],c1);patch([0 1 1 1-e 1-e 0+e],[0 0 1 1-e 0+e 0+e],c2);patch([0 0 1 1-e 0+e 0+e],[0 1 1 1-e 1-e 0+e],c3);plot([0 1 1 0 0],[0 0 1 1 0]);disp('Weights');
  "IW{1,1}(6,:)'" : Constant  Value=[0.87000976858961343030074431226239539682865142822265625;0.7110350945318122395377713473862968385219573974609375;-1.2759595695332432985225068478030152618885040283203125;1.2054218240237222214972234723973087966442108154296875;0.83833544909682855550414615208865143358707427978515625;1.5559780003582430740749487085849978029727935791015625;0.698202525683534691580689468537457287311553955078125;-0.17286948979518290681056669200188480317592620849609375;-0.373453768756931647754271352823707275092601776123046875]
      mask Display: e = 0.06;c1 = [120 150 230]/255;c2 = ([120 150 230]+0)/383;c3 = ([120 150 230]+128)/383;patch([0 1 1 0],[0 0 1 1],c1);patch([0 1 1 1-e 1-e 0+e],[0 0 1 1-e 0+e 0+e],c2);patch([0 0 1 1-e 0+e 0+e],[0 1 1 1-e 1-e 0+e],c3);plot([0 1 1 0 0],[0 0 1 1 0]);disp('Weights');
  "IW{1,1}(7,:)'" : Constant  Value=[1.4997372016747945178138934352318756282329559326171875;-0.418144995355191839703223877222626470029354095458984375;-0.223661784933861351731820832355879247188568115234375;0.9646418008850810021925781256868503987789154052734375;0.58275331566434107610774617569404654204845428466796875;1.4086511278745266206868791414308361709117889404296875;0.66061304729803682622701899163075722754001617431640625;-0.85347821356929298719506959969294257462024688720703125;0.564640016963342095124289699015207588672637939453125]
      mask Display: e = 0.06;c1 = [120 150 230]/255;c2 = ([120 150 230]+0)/383;c3 = ([120 150 230]+128)/383;patch([0 1 1 0],[0 0 1 1],c1);patch([0 1 1 1-e 1-e 0+e],[0 0 1 1-e 0+e 0+e],c2);patch([0 0 1 1-e 0+e 0+e],[0 1 1 1-e 1-e 0+e],c3);plot([0 1 1 0 0],[0 0 1 1 0]);disp('Weights');
  "IW{1,1}(8,:)'" : Constant  Value=[-0.64145815737887346141832267676363699138164520263671875;-1.1466409303196909430511141181341372430324554443359375;-0.376513844193542668303820164510398171842098236083984375;-0.354876733680442424390122369004529900848865509033203125;0.39032632476723494452386375996866263449192047119140625;1.1144230146539382264592177307349629700183868408203125;-0.99474015016140437950298291980288922786712646484375;1.34246851661036092906442718231119215488433837890625;-0.53861982069599945166515908567816950380802154541015625]
      mask Display: e = 0.06;c1 = [120 150 230]/255;c2 = ([120 150 230]+0)/383;c3 = ([120 150 230]+128)/383;patch([0 1 1 0],[0 0 1 1],c1);patch([0 1 1 1-e 1-e 0+e],[0 0 1 1-e 0+e 0+e],c2);patch([0 0 1 1-e 0+e 0+e],[0 1 1 1-e 1-e 0+e],c3);plot([0 1 1 0 0],[0 0 1 1 0]);disp('Weights');
  "IW{1,1}(9,:)'" : Constant  Value=[0.6499457547620723918413432329543866217136383056640625;0.87866119494201611050954170423210598528385162353515625;-1.01929567913466723183546491782180964946746826171875;-1.0428089589739835130188794209971092641353607177734375;0.68443113420214041209277411326183937489986419677734375;0.3412573356422889947481280614738352596759796142578125;0.59969312005255159814254284356138668954372406005859375;-1.1777031620542992573774654374574311077594757080078125;-0.96768538118119951096929298728355206549167633056640625]
      mask Display: e = 0.06;c1 = [120 150 230]/255;c2 = ([120 150 230]+0)/383;c3 = ([120 150 230]+128)/383;patch([0 1 1 0],[0 0 1 1],c1);patch([0 1 1 1-e 1-e 0+e],[0 0 1 1-e 0+e 0+e],c2);patch([0 0 1 1-e 0+e 0+e],[0 1 1 1-e 1-e 0+e],c3);plot([0 1 1 0 0],[0 0 1 1 0]);disp('Weights');
  Mux : Mux  Inputs=50
      mask Display: e = 0.06;c1 = [120 150 230]/255;c2 = ([120 150 230]+0)/383;c3 = ([120 150 230]+128)/383;patch([0 1 1 0],[0 0 1 1],c1);patch([0 1 1 1-e 1-e 0+e],[0 0 1 1-e 0+e 0+e],c2);patch([0 0 1 1-e 0+e 0+e],[0 1 1 1-e 1-e 0+e],c3);plot([0 1 1 0 0],[0 0 1 1 0]);disp('Mux');
  dotprod{1..50} (50 alike) : neural/Weight Functions/dotprod
  "iz{1,1}" : Outport
      mask Display: e = 0.06;c1 = [120 230 180]/255;c2 = ([120 230 180]+0)/(256+128);c3 = ([120 230 180]+128)/(256+128);patch([0 1 1 0],[0 0 1 1],c1);patch([0 1 1 1-e 1-e 0+e],[0 0 1 1-e 0+e 0+e],c2);patch([0 0 1 1-e 0+e 0+e],[0 1 1 1-e 1-e 0+e],c3);plot([0 1 1 0 0],[0 0 1 1 0]);
  wires:
  "IW{1,1}(1,:)'"/1 -> dotprod1/1
  "pd{1,1}"/1 -> dotprod1/2, dotprod2/2, dotprod3/2, dotprod4/2, dotprod5/2, dotprod6/2, dotprod7/2, dotprod8/2, dotprod9/2, dotprod10/2, dotprod11/2, dotprod12/2, dotprod13/2, dotprod14/2, dotprod15/2, dotprod16/2, dotprod17/2, dotprod18/2, dotprod19/2, dotprod20/2, dotprod21/2, dotprod22/2, dotprod23/2, dotprod24/2, dotprod25/2, dotprod26/2, dotprod27/2, dotprod28/2, dotprod29/2, dotprod30/2, dotprod31/2, dotprod32/2, dotprod33/2, dotprod34/2, dotprod35/2, dotprod36/2, dotprod37/2, dotprod38/2, dotprod39/2, dotprod40/2, dotprod41/2, dotprod42/2, dotprod43/2, dotprod44/2, dotprod45/2, dotprod46/2, dotprod47/2, dotprod48/2, dotprod49/2, dotprod50/2
  dotprod1/1 -> Mux/1
  "IW{1,1}(2,:)'"/1 -> dotprod2/1
  dotprod2/1 -> Mux/2
  "IW{1,1}(3,:)'"/1 -> dotprod3/1
  dotprod3/1 -> Mux/3
  "IW{1,1}(4,:)'"/1 -> dotprod4/1
  dotprod4/1 -> Mux/4
  "IW{1,1}(5,:)'"/1 -> dotprod5/1
  dotprod5/1 -> Mux/5
  "IW{1,1}(6,:)'"/1 -> dotprod6/1
  dotprod6/1 -> Mux/6
  "IW{1,1}(7,:)'"/1 -> dotprod7/1
  dotprod7/1 -> Mux/7
  "IW{1,1}(8,:)'"/1 -> dotprod8/1
  dotprod8/1 -> Mux/8
  "IW{1,1}(9,:)'"/1 -> dotprod9/1
  dotprod9/1 -> Mux/9
  "IW{1,1}(10,:)'"/1 -> dotprod10/1
  dotprod10/1 -> Mux/10
  "IW{1,1}(11,:)'"/1 -> dotprod11/1
  dotprod11/1 -> Mux/11
  "IW{1,1}(12,:)'"/1 -> dotprod12/1
  dotprod12/1 -> Mux/12
  "IW{1,1}(13,:)'"/1 -> dotprod13/1
  dotprod13/1 -> Mux/13
  "IW{1,1}(14,:)'"/1 -> dotprod14/1
  dotprod14/1 -> Mux/14
  "IW{1,1}(15,:)'"/1 -> dotprod15/1
  dotprod15/1 -> Mux/15
  "IW{1,1}(16,:)'"/1 -> dotprod16/1
  dotprod16/1 -> Mux/16
  "IW{1,1}(17,:)'"/1 -> dotprod17/1
  dotprod17/1 -> Mux/17
  "IW{1,1}(18,:)'"/1 -> dotprod18/1
  dotprod18/1 -> Mux/18
  "IW{1,1}(19,:)'"/1 -> dotprod19/1
  dotprod19/1 -> Mux/19
  "IW{1,1}(20,:)'"/1 -> dotprod20/1
  dotprod20/1 -> Mux/20
  "IW{1,1}(21,:)'"/1 -> dotprod21/1
  dotprod21/1 -> Mux/21
  "IW{1,1}(22,:)'"/1 -> dotprod22/1
  dotprod22/1 -> Mux/22
  "IW{1,1}(23,:)'"/1 -> dotprod23/1
  dotprod23/1 -> Mux/23
  "IW{1,1}(24,:)'"/1 -> dotprod24/1
  dotprod24/1 -> Mux/24
  "IW{1,1}(25,:)'"/1 -> dotprod25/1
  dotprod25/1 -> Mux/25
  "IW{1,1}(26,:)'"/1 -> dotprod26/1
  dotprod26/1 -> Mux/26
  "IW{1,1}(27,:)'"/1 -> dotprod27/1
  dotprod27/1 -> Mux/27
  "IW{1,1}(28,:)'"/1 -> dotprod28/1
  dotprod28/1 -> Mux/28
  "IW{1,1}(29,:)'"/1 -> dotprod29/1
  dotprod29/1 -> Mux/29
  "IW{1,1}(30,:)'"/1 -> dotprod30/1
  dotprod30/1 -> Mux/30
  "IW{1,1}(31,:)'"/1 -> dotprod31/1
  dotprod31/1 -> Mux/31
  "IW{1,1}(32,:)'"/1 -> dotprod32/1
  dotprod32/1 -> Mux/32
  "IW{1,1}(33,:)'"/1 -> dotprod33/1
  dotprod33/1 -> Mux/33
  "IW{1,1}(34,:)'"/1 -> dotprod34/1
  dotprod34/1 -> Mux/34
  "IW{1,1}(35,:)'"/1 -> dotprod35/1
  dotprod35/1 -> Mux/35
  "IW{1,1}(36,:)'"/1 -> dotprod36/1
  dotprod36/1 -> Mux/36
  "IW{1,1}(37,:)'"/1 -> dotprod37/1
  dotprod37/1 -> Mux/37
  "IW{1,1}(38,:)'"/1 -> dotprod38/1
  dotprod38/1 -> Mux/38
  "IW{1,1}(39,:)'"/1 -> dotprod39/1
  dotprod39/1 -> Mux/39
  "IW{1,1}(40,:)'"/1 -> dotprod40/1
  dotprod40/1 -> Mux/40
  "IW{1,1}(41,:)'"/1 -> dotprod41/1
  dotprod41/1 -> Mux/41
  "IW{1,1}(42,:)'"/1 -> dotprod42/1
  dotprod42/1 -> Mux/42
  "IW{1,1}(43,:)'"/1 -> dotprod43/1
  dotprod43/1 -> Mux/43
  "IW{1,1}(44,:)'"/1 -> dotprod44/1
  dotprod44/1 -> Mux/44
  "IW{1,1}(45,:)'"/1 -> dotprod45/1
  dotprod45/1 -> Mux/45
  "IW{1,1}(46,:)'"/1 -> dotprod46/1
  dotprod46/1 -> Mux/46
  "IW{1,1}(47,:)'"/1 -> dotprod47/1
  dotprod47/1 -> Mux/47
  "IW{1,1}(48,:)'"/1 -> dotprod48/1
  dotprod48/1 -> Mux/48
  "IW{1,1}(49,:)'"/1 -> dotprod49/1
  dotprod49/1 -> Mux/49
  "IW{1,1}(50,:)'"/1 -> dotprod50/1
  dotprod50/1 -> Mux/50
  Mux/1 -> "iz{1,1}"/1

== system control_system/Function Fitting Neural Network/Layer 2/Delays 1 ==
  "p{2}" : Inport  PortDimensions=50  SampleTime=0.1
      mask Display: e = 0.06;c1 = [120 230 180]/255;c2 = ([120 230 180]+0)/(256+128);c3 = ([120 230 180]+128)/(256+128);patch([0 1 1 0],[0 0 1 1],c1);patch([0 1 1 1-e 1-e 0+e],[0 0 1 1-e 0+e 0+e],c2);patch([0 0 1 1-e 0+e 0+e],[0 1 1 1-e 1-e 0+e],c3);plot([0 1 1 0 0],[0 0 1 1 0]);
  mux : Mux  Inputs=1
      mask Display: e = 0.06;c1 = [120 150 230]/255;c2 = ([120 150 230]+0)/383;c3 = ([120 150 230]+128)/383;patch([0 1 1 0],[0 0 1 1],c1);patch([0 1 1 1-e 1-e 0+e],[0 0 1 1-e 0+e 0+e],c2);patch([0 0 1 1-e 0+e 0+e],[0 1 1 1-e 1-e 0+e],c3);plot([0 1 1 0 0],[0 0 1 1 0]);disp('Mux')
  "pd{2,1}" : Outport
      mask Display: e = 0.06;c1 = [120 230 180]/255;c2 = ([120 230 180]+0)/(256+128);c3 = ([120 230 180]+128)/(256+128);patch([0 1 1 0],[0 0 1 1],c1);patch([0 1 1 1-e 1-e 0+e],[0 0 1 1-e 0+e 0+e],c2);patch([0 0 1 1-e 0+e 0+e],[0 1 1 1-e 1-e 0+e],c3);plot([0 1 1 0 0],[0 0 1 1 0]);
  wires:
  "p{2}"/1 -> mux/1
  mux/1 -> "pd{2,1}"/1
